simulink model "Pendulum"  (R2022b)
settings: Solver=VariableStepAuto  StartTime=0.0  StopTime=20  RelTol=1e-3
values from neighbouring files (symbols this model uses):
  F = lqr(A,B,Q,R)    [startup.m]
  g = 9.81    [startup.m]
  I = 1/3*m*L^2    (= 2.743875)    [startup.m]
  Lc = L/2    (= 0.75)    [startup.m]
  m = L*(0.03)*(0.03)*rho_aluminum    (= 3.6585)    [startup.m]
  q_0 = deg2rad(-80)    [startup.m]
undefined symbols (not defined in the file or in its folder): I1, I2, L1, Lc1, Lc2, m1, m2, q1_0, q2_0
settings Model: Creator=logan  LastModifiedBy=logan

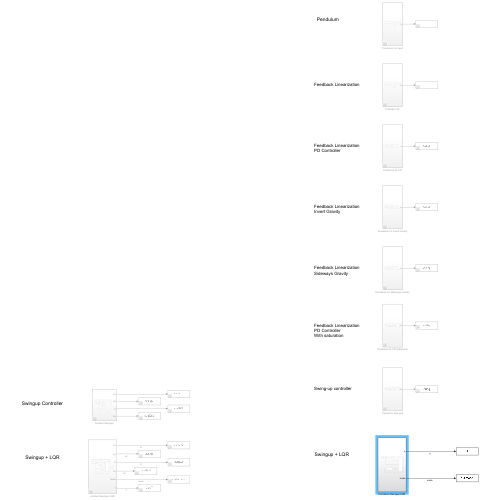
[thumbnail: Simulink's stored preview of the top-level diagram]
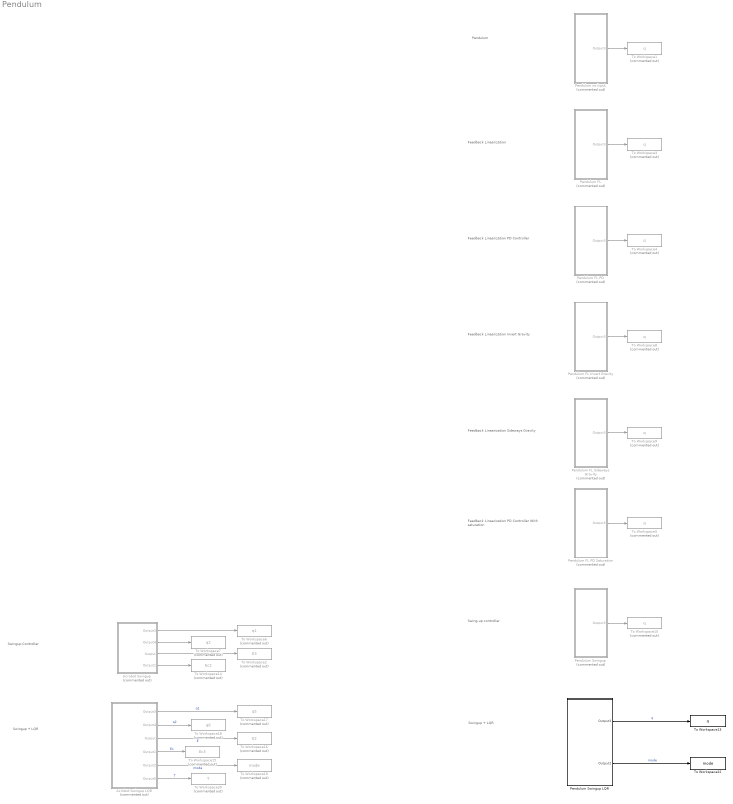
== system Pendulum ==
  note: Feedback Linearization
  note: Swingup Controller
  note: Swingup + LQR
  note: Pendulum
  note: Feedback Linearization
      | PD Controller
  note: Feedback Linearization
      | PD Controller
      | With saturation
  note: Feedback Linearization
      | Invert Gravity
  note: Feedback Linearization
      | Sideways Gravity
  note: Swing-up controller
  note: Swingup + LQR
  Acrobot Swingup : Subsystem  Commented=on
  Acrobot Swingup LQR : Subsystem  Commented=on
  Pendulum FL : Subsystem  Commented=on
  Pendulum FL Invert Gravity : Subsystem  Commented=on
  Pendulum FL PD : Subsystem  Commented=on
  Pendulum FL PD Saturation : Subsystem  Commented=on
  Pendulum FL Sideways Gravity : Subsystem  Commented=on
  Pendulum Swingup : Subsystem  Commented=on
  Pendulum Swingup LQR : Subsystem
  Pendulum no input : Subsystem  Commented=on
  To Workspace{1,3..5,8..10} (7 alike) : ToWorkspace  Commented=on  VariableName=q  SaveFormat=Timeseries  SampleTime=-1
  To Workspace13 : ToWorkspace  VariableName=q  SaveFormat=Timeseries  SampleTime=-1
  To Workspace14 : ToWorkspace  Commented=on  VariableName=Ec2  SaveFormat=Timeseries  SampleTime=-1
  To Workspace15 : ToWorkspace  Commented=on  VariableName=Ec3  SaveFormat=Timeseries  SampleTime=-1
  To Workspace16 : ToWorkspace  Commented=on  VariableName=E2  SaveFormat=Timeseries  SampleTime=-1
  To Workspace17 : ToWorkspace  Commented=on  VariableName=q5  SaveFormat=Timeseries  SampleTime=-1
  To Workspace18 : ToWorkspace  Commented=on  VariableName=q6  SaveFormat=Timeseries  SampleTime=-1
  To Workspace19 : ToWorkspace  Commented=on  VariableName=mode  SaveFormat=Timeseries  SampleTime=-1
  To Workspace2 : ToWorkspace  Commented=on  VariableName=E3  SaveFormat=Timeseries  SampleTime=-1
  To Workspace20 : ToWorkspace  Commented=on  VariableName=T  SaveFormat=Timeseries  SampleTime=-1
  To Workspace22 : ToWorkspace  VariableName=mode  SaveFormat=Timeseries  SampleTime=-1
  To Workspace6 : ToWorkspace  Commented=on  VariableName=q1  SaveFormat=Timeseries  SampleTime=-1
  To Workspace7 : ToWorkspace  Commented=on  VariableName=q2  SaveFormat=Timeseries  SampleTime=-1
  wires:
  Acrobot Swingup LQR/6(Output5) -> To Workspace20/1  "T"
  Acrobot Swingup LQR/5(Output2) -> To Workspace19/1  "mode"
  Acrobot Swingup/1(Output3) -> To Workspace6/1
  Acrobot Swingup LQR/4(Output1) -> To Workspace15/1  "Ec"
  Acrobot Swingup LQR/1(Output3) -> To Workspace17/1  "q1"
  Acrobot Swingup LQR/2(Output4) -> To Workspace18/1  "q2"
  Acrobot Swingup/3(Output) -> To Workspace2/1
  Acrobot Swingup/4(Output1) -> To Workspace14/1
  Acrobot Swingup LQR/3(Output) -> To Workspace16/1  "E"
  Acrobot Swingup/2(Output4) -> To Workspace7/1
  Pendulum no input/1(Output3) -> To Workspace1/1
  Pendulum FL/1(Output3) -> To Workspace3/1
  Pendulum FL PD/1(Output3) -> To Workspace4/1
  Pendulum FL PD Saturation/1(Output3) -> To Workspace5/1
  Pendulum FL Invert Gravity/1(Output3) -> To Workspace8/1
  Pendulum FL Sideways Gravity/1(Output3) -> To Workspace9/1
  Pendulum Swingup/1(Output3) -> To Workspace10/1
  Pendulum Swingup LQR/1(Output3) -> To Workspace13/1  "q"
  Pendulum Swingup LQR/2(Output2) -> To Workspace22/1  "mode"

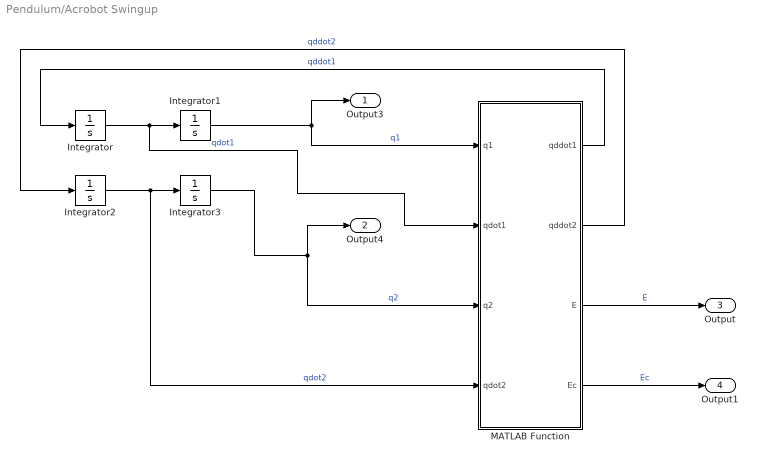
== system Pendulum/Acrobot Swingup ==
  Integrator : Integrator
  Integrator1 : Integrator  InitialCondition=q1_0
  Integrator2 : Integrator
  Integrator3 : Integrator  InitialCondition=q2_0
  MATLAB Function : MATLAB Function  TreatAsAtomicUnit=on
  Output3 : Outport
  Output4 : Outport  Port=2
  Output : Outport  Port=3
  Output1 : Outport  Port=4
  wires:
  Integrator/1 -> MATLAB Function/2(qdot1), Integrator1/1  "qdot1"
  Integrator1/1 -> Output3/1, MATLAB Function/1(q1)  "q1"
  Integrator2/1 -> MATLAB Function/4(qdot2), Integrator3/1  "qdot2"
  MATLAB Function/2(qddot2) -> Integrator2/1  "qddot2"
  Integrator3/1 -> Output4/1, MATLAB Function/3(q2)  "q2"
  MATLAB Function/1(qddot1) -> Integrator/1  "qddot1"
  MATLAB Function/3(E) -> Output/1  "E"
  MATLAB Function/4(Ec) -> Output1/1  "Ec"

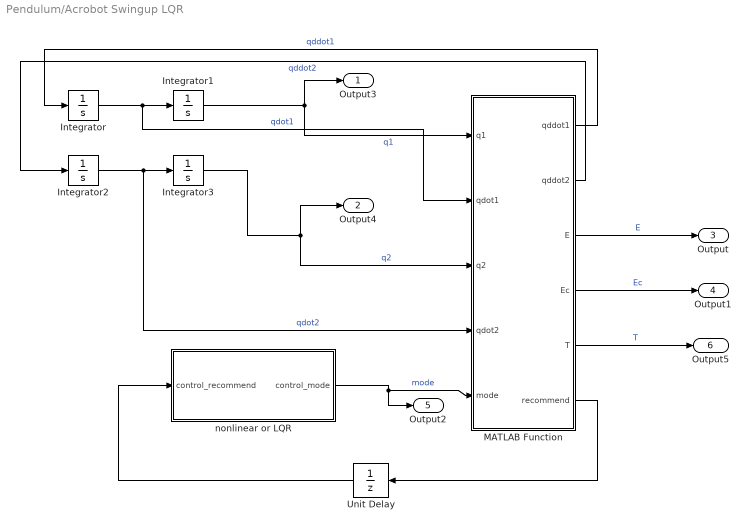
== system Pendulum/Acrobot Swingup LQR ==
  Integrator : Integrator
  Integrator1 : Integrator  InitialCondition=q1_0
  Integrator2 : Integrator
  Integrator3 : Integrator  InitialCondition=q2_0
  MATLAB Function : MATLAB Function  TreatAsAtomicUnit=on
  Unit Delay : UnitDelay  SampleTime=1/30  HasFrameUpgradeWarning=on
  nonlinear or LQR : Stateflow chart  TreatAsAtomicUnit=on
  Output3 : Outport
  Output4 : Outport  Port=2
  Output : Outport  Port=3
  Output1 : Outport  Port=4
  Output2 : Outport  Port=5
  Output5 : Outport  Port=6
  wires:
  Integrator/1 -> MATLAB Function/2(qdot1), Integrator1/1  "qdot1"
  Integrator1/1 -> Output3/1, MATLAB Function/1(q1)  "q1"
  Integrator2/1 -> MATLAB Function/4(qdot2), Integrator3/1  "qdot2"
  MATLAB Function/2(qddot2) -> Integrator2/1  "qddot2"
  Integrator3/1 -> Output4/1, MATLAB Function/3(q2)  "q2"
  MATLAB Function/1(qddot1) -> Integrator/1  "qddot1"
  MATLAB Function/3(E) -> Output/1  "E"
  MATLAB Function/4(Ec) -> Output1/1  "Ec"
  nonlinear or LQR/1(control_mode) -> Output2/1, MATLAB Function/5(mode)  "mode"
  MATLAB Function/6(recommend) -> Unit Delay/1
  Unit Delay/1 -> nonlinear or LQR/1(control_recommend)
  MATLAB Function/5(T) -> Output5/1  "T"

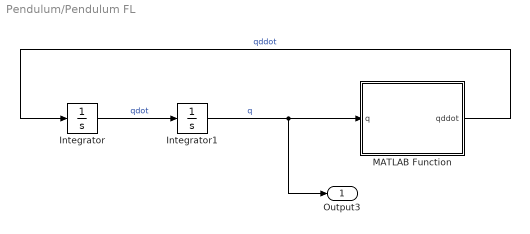
== system Pendulum/Pendulum FL ==
  Integrator : Integrator
  Integrator1 : Integrator  InitialCondition=q_0
  MATLAB Function : MATLAB Function  TreatAsAtomicUnit=on
  Output3 : Outport
  wires:
  Integrator/1 -> Integrator1/1  "qdot"
  MATLAB Function/1(qddot) -> Integrator/1  "qddot"
  Integrator1/1 -> Output3/1, MATLAB Function/1(q)  "q"

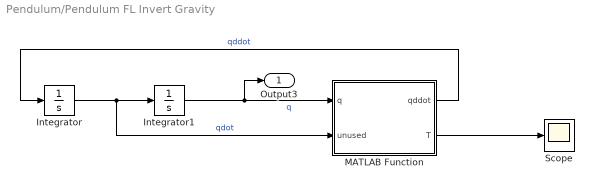
== system Pendulum/Pendulum FL Invert Gravity ==
  Integrator : Integrator
  Integrator1 : Integrator  InitialCondition=q_0
  MATLAB Function : MATLAB Function  TreatAsAtomicUnit=on
  Scope : Scope
  Output3 : Outport
  wires:
  Integrator/1 -> MATLAB Function/2(unused), Integrator1/1  "qdot"
  MATLAB Function/1(qddot) -> Integrator/1  "qddot"
  Integrator1/1 -> Output3/1, MATLAB Function/1(q)  "q"
  MATLAB Function/2(T) -> Scope/1

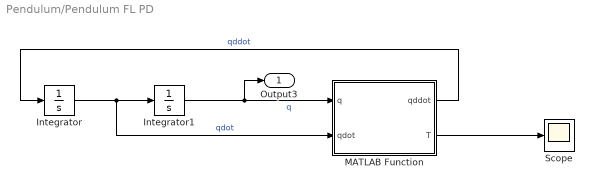
== system Pendulum/Pendulum FL PD ==
  Integrator : Integrator
  Integrator1 : Integrator  InitialCondition=-pi/2
  MATLAB Function : MATLAB Function  TreatAsAtomicUnit=on
  Scope : Scope
  Output3 : Outport
  wires:
  Integrator/1 -> MATLAB Function/2(qdot), Integrator1/1  "qdot"
  MATLAB Function/1(qddot) -> Integrator/1  "qddot"
  Integrator1/1 -> Output3/1, MATLAB Function/1(q)  "q"
  MATLAB Function/2(T) -> Scope/1

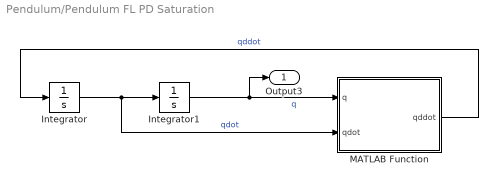
== system Pendulum/Pendulum FL PD Saturation ==
  Integrator : Integrator
  Integrator1 : Integrator  InitialCondition=-pi/2
  MATLAB Function : MATLAB Function  TreatAsAtomicUnit=on
  Output3 : Outport
  wires:
  Integrator/1 -> MATLAB Function/2(qdot), Integrator1/1  "qdot"
  MATLAB Function/1(qddot) -> Integrator/1  "qddot"
  Integrator1/1 -> Output3/1, MATLAB Function/1(q)  "q"

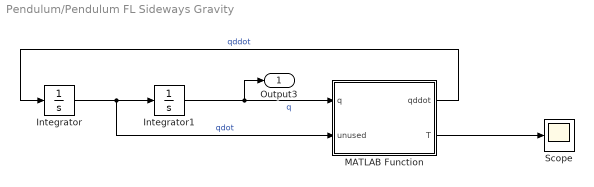
== system Pendulum/Pendulum FL Sideways Gravity ==
  Integrator : Integrator
  Integrator1 : Integrator  InitialCondition=q_0
  MATLAB Function : MATLAB Function  TreatAsAtomicUnit=on
  Scope : Scope
  Output3 : Outport
  wires:
  Integrator/1 -> MATLAB Function/2(unused), Integrator1/1  "qdot"
  MATLAB Function/1(qddot) -> Integrator/1  "qddot"
  Integrator1/1 -> Output3/1, MATLAB Function/1(q)  "q"
  MATLAB Function/2(T) -> Scope/1

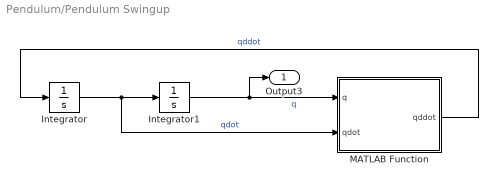
== system Pendulum/Pendulum Swingup ==
  Integrator : Integrator
  Integrator1 : Integrator  InitialCondition=q_0
  MATLAB Function : MATLAB Function  TreatAsAtomicUnit=on
  Output3 : Outport
  wires:
  Integrator/1 -> MATLAB Function/2(qdot), Integrator1/1  "qdot"
  MATLAB Function/1(qddot) -> Integrator/1  "qddot"
  Integrator1/1 -> Output3/1, MATLAB Function/1(q)  "q"

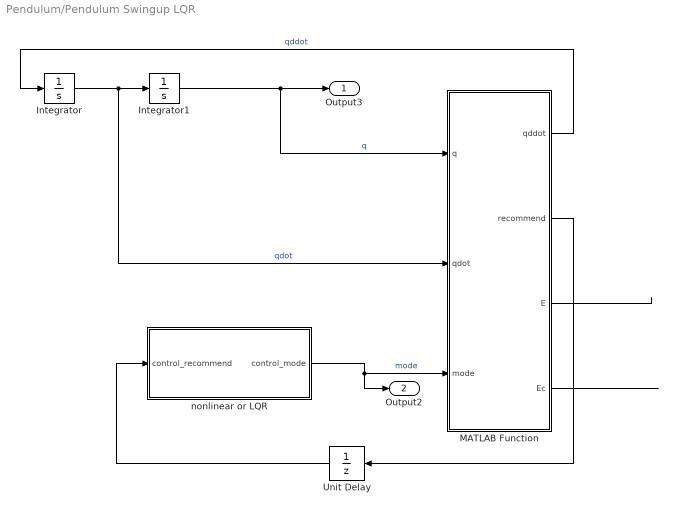
== system Pendulum/Pendulum Swingup LQR ==
  Integrator : Integrator
  Integrator1 : Integrator  InitialCondition=q_0
  MATLAB Function : MATLAB Function  TreatAsAtomicUnit=on
  Unit Delay : UnitDelay  SampleTime=1/30  HasFrameUpgradeWarning=on
  nonlinear or LQR : Stateflow chart  TreatAsAtomicUnit=on
  Output3 : Outport
  Output2 : Outport  Port=2
  wires:
  Integrator/1 -> MATLAB Function/2(qdot), Integrator1/1  "qdot"
  Integrator1/1 -> Output3/1, MATLAB Function/1(q)  "q"
  MATLAB Function/1(qddot) -> Integrator/1  "qddot"
  nonlinear or LQR/1(control_mode) -> Output2/1, MATLAB Function/3(mode)  "mode"
  MATLAB Function/2(recommend) -> Unit Delay/1
  Unit Delay/1 -> nonlinear or LQR/1(control_recommend)
  MATLAB Function/3(E) -> ?
  MATLAB Function/4(Ec) -> ?

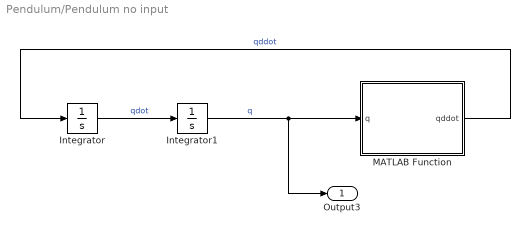
== system Pendulum/Pendulum no input ==
  Integrator : Integrator
  Integrator1 : Integrator  InitialCondition=q_0
  MATLAB Function : MATLAB Function  TreatAsAtomicUnit=on
  Output3 : Outport
  wires:
  Integrator/1 -> Integrator1/1  "qdot"
  MATLAB Function/1(qddot) -> Integrator/1  "qddot"
  Integrator1/1 -> Output3/1, MATLAB Function/1(q)  "q"

== matlab function Pendulum/Acrobot Swingup/MATLAB Function ==
  data: q1 input; qdot1 input; q2 input; qdot2 input; qddot1 output; qddot2 output; g parameter; I2 parameter; Lc2 parameter; m2 parameter; I1 parameter; Lc1 parameter; L1 parameter; m1 parameter; E output; Ec output
function [qddot1,qddot2,E,Ec] = ...
    EoM(q1,qdot1,q2,qdot2,g, I2, Lc2, m2, I1, Lc1, L1, m1)

m11 = m1*Lc1^2 + m2*(L1^2 + Lc2^2 + 2*L1*Lc2*cos(q2)) + I1 + I2;
m12 = m2*(Lc2^2 + L1*Lc2*cos(q2)) + I2;
m22 = m2*Lc2^2 + I2;

h1 = -m2*L1*Lc2*sin(q2)*qdot2^2 - 2*m2*L1*Lc2*sin(q2)*qdot2*qdot1;
phi1 = (m1*Lc1+m2*L1)*g*cos(q1) + m2*Lc2*g*cos(q1+q2);

% energy calculations
yc1 = Lc1*sin(q1);
yc2 = L1*sin(q1) + Lc2*sin(q1+q2);K = 0.5*m11*qdot1^2 + m12*qdot1*qdot2 + 0.5*m22*qdot2^2;
P = g*(m1*yc1 + m2*yc2);
E = K + P;
Ec = g*(m1*Lc1 + m2*(L1+Lc2)); % upright potential energy

% equations of motion (PFL)
% with pole placement
% and nonlinear swingup control
k2 = 10;
k1 = 21;

u_bar = (Ec-E)*qdot1;
sat_ubar = min(10, max(-10, u_bar));
% sat_ubar = u_bar;

u = sat_ubar - k2*qdot2 - k1*q2;
qddot2 = u;
qddot1 = -1/m11*(m12*u + h1 + phi1);

== matlab function Pendulum/Pendulum FL PD Saturation/MATLAB Function ==
  data: q input; qdot input; g parameter; qddot output; m parameter; I parameter; Lc parameter
function qddot  = EoM(q,qdot,g,m,I,Lc)

% feedback linearization w/ PD controller
u = -10*qdot - 21*(q-pi/2);
T = I*u + m*g*Lc*cos(q);

% saturation
T = min(15, max(-15, T));

% dynamics (cannot get to equilibrium point)
qddot = 1/I*(-m*g*Lc*cos(q) + T);

== stateflow chart Pendulum/Acrobot Swingup LQR/nonlinear or LQR ==
  state nonlinear
    control_mode=1;
  state LQR
    control_mode=2;
  (default) -> nonlinear
  nonlinear -> LQR : [control_recommend==2]
  data: control_recommend input; control_mode output

== matlab function Pendulum/Pendulum FL Invert Gravity/MATLAB Function ==
  data: q input; unused input; g parameter; qddot output; m parameter; I parameter; Lc parameter; T output
function [qddot,T]  = EoM(q,~,g,m,I,Lc)

% feedback linearization w/ PD controller
u = 1/I*(m*g*Lc*cos(q));
T = I*u + m*g*Lc*cos(q);

% dynamics
qddot = 1/I*(-m*g*Lc*cos(q) + T);

== matlab function Pendulum/Pendulum FL Sideways Gravity/MATLAB Function ==
  data: q input; unused input; g parameter; qddot output; m parameter; I parameter; Lc parameter; T output
function [qddot,T]  = EoM(q,~,g,m,I,Lc)

% feedback linearization w/ PD controller
u = -1/I*(m*g*Lc*sin(q));
T = I*u + m*g*Lc*cos(q);

% dynamics
qddot = 1/I*(-m*g*Lc*cos(q) + T);

== matlab function Pendulum/Pendulum Swingup/MATLAB Function ==
  data: q input; qdot input; g parameter; qddot output; m parameter; I parameter; Lc parameter
function qddot  = EoM(q,qdot,g,m,I,Lc)

% swing-up controller
E = 1/2*I*qdot^2 + m*g*Lc*sin(q);
Ec = m*g*Lc*sin(pi/2);

T = (Ec-E)*qdot;

% saturation
T = min(5, max(-5, T));

% dynamics
qddot = 1/I*(-m*g*Lc*cos(q) + T);

== matlab function Pendulum/Pendulum Swingup LQR/MATLAB Function ==
  data: q input; qdot input; mode input; g parameter; qddot output; Lc parameter; recommend output; I parameter; m parameter; F parameter; E output; Ec output
function [qddot,recommend,E,Ec]  = EoM(q,qdot,mode,g,Lc,I,m,F)

% swing-up controller
E = 1/2*I*qdot^2 + m*g*Lc*sin(q);
Ec = m*g*Lc*sin(pi/2);
T_nonlinear = (Ec-E)*qdot;

% LQR controller
z = wrapToPi(q)-pi/2;
T_lqr = -F*[z; qdot];

if mode == 1
    T = T_nonlinear;
else
    T = T_lqr;
end

% saturation
T = min(5, max(-5, T));

% dynamics
qddot = 1/I*(-m*g*Lc*cos(q) + T);

% starts in nonlinear mode, switches to LQR at the right moment
% does not switch back to nonlinear mode once we are in LQR
if abs(z) < deg2rad(5)
    recommend = 2; % LQR
else
    recommend = 1; % nonlinear
end

== stateflow chart Pendulum/Pendulum Swingup LQR/nonlinear or LQR ==
  state nonlinear
    control_mode=1;
  state LQR
    control_mode=2;
  (default) -> nonlinear
  nonlinear -> LQR : [control_recommend==2]
  data: control_recommend input; control_mode output

== matlab function Pendulum/Acrobot Swingup LQR/MATLAB Function ==
  data: q1 input; qdot1 input; q2 input; qdot2 input; mode input; qddot1 output; qddot2 output; g parameter; I2 parameter; Lc2 parameter; m2 parameter; I1 parameter; Lc1 parameter; L1 parameter; m1 parameter; E output; Ec output; T output; F parameter; recommend output
function [qddot1,qddot2,E,Ec,T,recommend] = ...
    EoM(q1,qdot1,q2,qdot2,mode,g,I2,Lc2,m2,I1,Lc1,L1,m1,F)

% equations of motion
m11 = m1*Lc1^2 + m2*(L1^2 + Lc2^2 + 2*L1*Lc2*cos(q2)) + I1 + I2;
m12 = m2*(Lc2^2 + L1*Lc2*cos(q2)) + I2;
m22 = m2*Lc2^2 + I2;

h1 = -m2*L1*Lc2*sin(q2)*qdot2^2 - 2*m2*L1*Lc2*sin(q2)*qdot2*qdot1;
h2 = m2*L1*Lc2*sin(q2)*qdot1^2;

phi1 = (m1*Lc1+m2*L1)*g*cos(q1) + m2*Lc2*g*cos(q1+q2);
phi2 = m2*Lc2*g*cos(q1+q2);

m22_bar = m22 - m12^2/m11;
h2_bar = h2 - m12*h1/m11;
phi2_bar = phi2 - m12*phi1/m11;

% energy calculations
yc1 = Lc1*sin(q1);
yc2 = L1*sin(q1) + Lc2*sin(q1+q2);
K = 0.5*m11*qdot1^2 + m12*qdot1*qdot2 + 0.5*m22*qdot2^2;
P = g*(m1*yc1 + m2*yc2);
E = K + P;
Ec = g*(m1*Lc1 + m2*(L1+Lc2)); % upright potential energy

% equations of motion (PFL)
% with pole placement
% and nonlinear swingup control
k2 = 10;
k1 = 21;

u_bar = (Ec-E)*qdot1;
u_nonlinear = u_bar - k2*qdot2 - k1*q2;
T_nonlinear = m22_bar*u_nonlinear + h2_bar + phi2_bar;

% LQR (accounting for non-zero set point)
z1 = wrapToPi(q1)-pi/2;
z2 = wrapToPi(q2);
T_lqr = -F*[z1; z2; qdot1; qdot2];

% dynamics
if mode == 1
    T = T_nonlinear;
else
    T = T_lqr;
end

% saturation
T = min(25, max(-25, T));
qddot2 = 1/m22_bar*(T - h2_bar - phi2_bar);
qddot1 = -1/m11*(m12*qddot2 + h1 + phi1);


% starts in nonlinear mode, switches to LQR at the right moment
% does not switch back to nonlinear mode once we are in LQR
if abs(z1) < deg2rad(5)
    recommend = 2; % LQR
else
    recommend = 1; % nonlinear
end

== matlab function Pendulum/Pendulum no input/MATLAB Function ==
  data: q input; g parameter; qddot output; m parameter; I parameter; Lc parameter
function qddot  = EoM(q,g,m,I,Lc)

T = 0; % input torque
qddot = 1/I*(-m*g*Lc*cos(q) + T);

== matlab function Pendulum/Pendulum FL PD/MATLAB Function ==
  data: q input; qdot input; g parameter; qddot output; m parameter; I parameter; Lc parameter; T output
function [qddot,T]  = EoM(q,qdot,g,m,I,Lc)

% feedback linearization w/ PD controller
u = -10*qdot - 21*(q-pi/2);
T = I*u + m*g*Lc*cos(q);

% dynamics
qddot = 1/I*(-m*g*Lc*cos(q) + T);

== matlab function Pendulum/Pendulum FL/MATLAB Function ==
  data: q input; g parameter; qddot output; m parameter; I parameter; Lc parameter
function qddot  = EoM(q,g,m,I,Lc)

% feedback linearization
u = 0;
T = I*u + m*g*Lc*cos(q); 

% dynamics
qddot = 1/I*(-m*g*Lc*cos(q) + T);
